simulink model "Week3_Q2"  (R2020b)
settings: Solver=FixedStepAuto  StartTime=0.0  StopTime=200  FixedStep=0.1  RelTol=1e-3
undefined symbols (not defined in the file): DiscIntNeverNeededParam
libraries: simulink x1
settings Model: Creator=DELL  LastModifiedBy=DELL

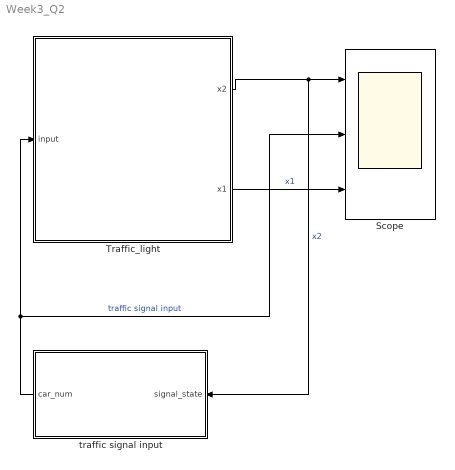
== system Week3_Q2 ==
  Scope : Scope  NumInputPorts=3
  Traffic_light : Stateflow chart  TreatAsAtomicUnit=on
  traffic signal input : Subsystem
  wires:
  traffic signal input/1(car_num) -> Scope/2, Traffic_light/1(input)  "traffic signal input"
  Traffic_light/1(x2) -> traffic signal input/1(signal_state), Scope/1  "x2"
  Traffic_light/2(x1) -> Scope/3  "x1"

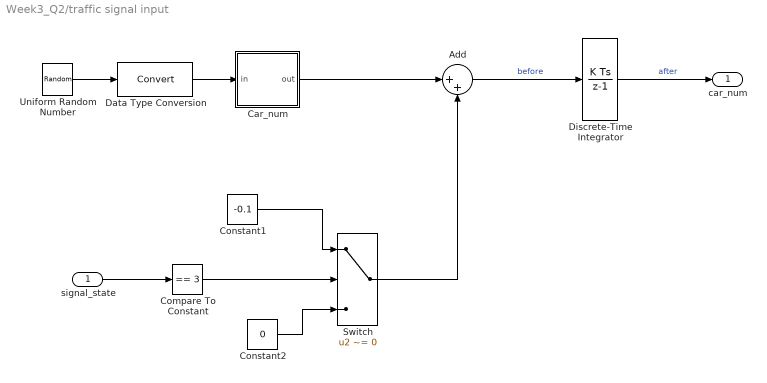
== system Week3_Q2/traffic signal input ==
  signal_state : Inport
  Add : Sum  Inputs=|++
  Car_num : Stateflow chart  TreatAsAtomicUnit=on
  Compare To Constant : simulink/Logic and Bit Operations/Compare To Constant  relop===  const=3  OutDataTypeStr=boolean  ZeroCross=off
  Constant1 : Constant  Value=-0.1
  Constant2 : Constant  Value=0
  Data Type Conversion : DataTypeConversion
  Discrete-Time Integrator : DiscreteIntegrator  SampleTime=-1  LimitOutput=on  LowerSaturationLimit=0  ICPrevOutput=DiscIntNeverNeededParam  ICPrevScaledInput=DiscIntNeverNeededParam
  Switch : Switch  Criteria=u2 ~= 0
  Uniform Random Number : UniformRandomNumber  Minimum=0  Maximum=100  Seed=177836  SampleTime=0
  car_num : Outport  VectorParamsAs1DForOutWhenUnconnected=off
  wires:
  Constant1/1 -> Switch/1
  Constant2/1 -> Switch/3
  Discrete-Time Integrator/1 -> car_num/1  "after"
  signal_state/1 -> Compare To Constant/1
  Compare To Constant/1 -> Switch/2
  Switch/1 -> Add/2
  Add/1 -> Discrete-Time Integrator/1  "before"
  Car_num/1(out) -> Add/1
  Data Type Conversion/1 -> Car_num/1(in)
  Uniform Random Number/1 -> Data Type Conversion/1

== stateflow chart Week3_Q2/Traffic_light ==
  state Stop
    entry:
    x1 = RED;
    x2 = GREEN;
  state Transition1
    entry:
    x1 = RED;
    x2 = YELLOW;
  state Initial
    entry:
    x1 = RED;
    x2 = GREEN;
  state Transition2
    entry:
    x1 = YELLOW;
    x2 = RED;
  state Go
    entry:
    x1 = GREEN;
    x2 = RED;
  (default) -> Initial
  Initial -> Stop : after(10,tick)
  Stop -> Transition1 : [input]
  Transition1 -> Go : after(3,tick)
  Transition2 -> Initial : after(3,tick)
  Go -> Transition2 : after(5,tick)
  data: GREEN constant double =3; RED constant double =1; YELLOW constant double =2; x2 output; x1 output; input input

== stateflow chart Week3_Q2/traffic signal input/Car_num ==
  (default) -> (junction 2) : {out = in > 98;}
  data: in input int8; out output double
